simulink model "test_attcontrol"  (R2020b)
settings: Solver=FixedStepAuto  StartTime=0.0  StopTime=N-1  FixedStep=time_step  RelTol=1e-3
values from neighbouring files (symbols this model uses):
  dw_rdt = ones(N,1)    [AttitudeControlTesting.m]
  m_mag = ones(N,1)*[1 1 1]/sqrt(3)    [AttitudeControlTesting.m]
  q_sc = [ones(N/2,1)*[0 0 0 1] ; ones(N/2,1)*[0 sin(pi/4) 0 cos(pi/4)] ]    [AttitudeControlTesting.m]
  time_step = 1    [AttitudeControlTesting.m]    (also in StateTesting.m)
  w_sc = ones(N,1)*deg2rad([0 0 1])    [AttitudeControlTesting.m]
  wr0 = 0    [AttitudeControlTesting.m]
undefined symbols (not defined in the file or in its folder): sim_constants
libraries: vrlib x3
settings Model: Creator=newpo  LastModifiedBy=newpo
settings DataIOCC: ReturnWorkspaceOutputs=off

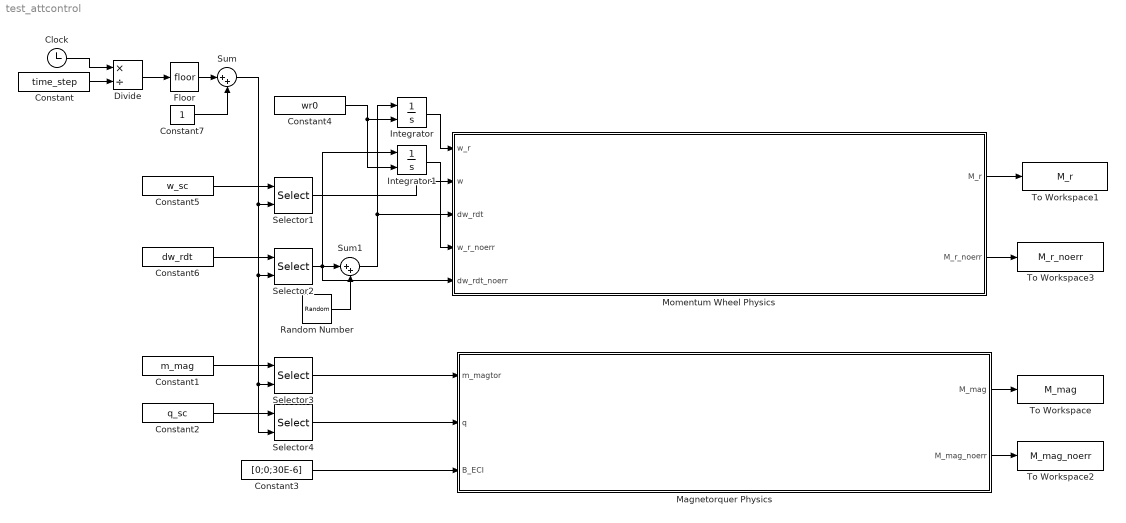
== system test_attcontrol ==
  Clock : Clock
  Constant : Constant  Value=time_step
  Constant1 : Constant  Value=m_mag
  Constant2 : Constant  Value=q_sc
  Constant3 : Constant  Value=[0;0;30E-6]
  Constant4 : Constant  Value=wr0
  Constant5 : Constant  Value=w_sc
  Constant6 : Constant  Value=dw_rdt
  Constant7 : Constant
  Divide : Product  Inputs=*/
  Floor : Rounding
  Integrator : Integrator  InitialConditionSource=external
  Integrator1 : Integrator  InitialConditionSource=external
  Magnetorquer Physics : Subsystem
  Momentum Wheel Physics : Subsystem
  Random Number : RandomNumber  Mean=sim_constants.dw_rdt_bias  Variance=sim_constants.dw_rdt_err  Seed=1  SampleTime=time_step  VectorParams1D=off
  Selector1 : Selector  NumberOfDimensions=2  InputPortWidth=3  IndexOptions=Index vector (port),Index vector (dialog)  Indices=[1 3],[1 2 3]  OutputSizes=1,1
  Selector2 : Selector  InputPortWidth=N  IndexOptions=Index vector (port)  Indices=[1 3]  OutputSizes=1
  Selector3 : Selector  NumberOfDimensions=2  InputPortWidth=3  IndexOptions=Index vector (port),Index vector (dialog)  Indices=[1 3],[1 2 3]  OutputSizes=1,1
  Selector4 : Selector  NumberOfDimensions=2  InputPortWidth=3  IndexOptions=Index vector (port),Index vector (dialog)  Indices=[1 3],[1 2 3 4]  OutputSizes=1,1
  Sum : Sum  Inputs=|++
  Sum1 : Sum  Inputs=|++
  To Workspace : ToWorkspace  VariableName=M_mag  SaveFormat=Timeseries  SampleTime=-1
  To Workspace1 : ToWorkspace  VariableName=M_r  SaveFormat=Timeseries  SampleTime=-1
  To Workspace2 : ToWorkspace  VariableName=M_mag_noerr  SaveFormat=Timeseries  SampleTime=-1
  To Workspace3 : ToWorkspace  VariableName=M_r_noerr  SaveFormat=Timeseries  SampleTime=-1
  wires:
  Selector1/1 -> Momentum Wheel Physics/2(w)
  Constant5/1 -> Selector1/1
  Sum1/1 -> Integrator/1, Momentum Wheel Physics/3(dw_rdt)
  Floor/1 -> Sum/1
  Sum/1 -> Selector4/2, Selector3/2, Selector2/2, Selector1/2
  Constant/1 -> Divide/2
  Clock/1 -> Divide/1
  Divide/1 -> Floor/1
  Constant7/1 -> Sum/2
  Constant6/1 -> Selector2/1
  Integrator/1 -> Momentum Wheel Physics/1(w_r)
  Constant4/1 -> Integrator1/2, Integrator/2
  Selector3/1 -> Magnetorquer Physics/1(m_magtor)
  Constant1/1 -> Selector3/1
  Selector4/1 -> Magnetorquer Physics/2(q)
  Constant2/1 -> Selector4/1
  Constant3/1 -> Magnetorquer Physics/3(B_ECI)
  Magnetorquer Physics/1(M_mag) -> To Workspace/1
  Momentum Wheel Physics/1(M_r) -> To Workspace1/1
  Magnetorquer Physics/2(M_mag_noerr) -> To Workspace2/1
  Momentum Wheel Physics/2(M_r_noerr) -> To Workspace3/1
  Selector2/1 -> Momentum Wheel Physics/5(dw_rdt_noerr), Integrator1/1, Sum1/1
  Random Number/1 -> Sum1/2
  Integrator1/1 -> Momentum Wheel Physics/4(w_r_noerr)

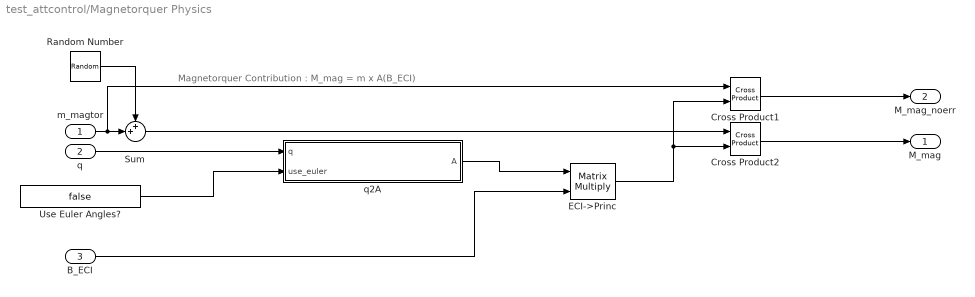
== system test_attcontrol/Magnetorquer Physics ==
  note: Magnetorquer Contribution : M_mag = m x A(B_ECI)
  m_magtor : Inport
  q : Inport  Port=2
  B_ECI : Inport  Port=3
  Cross Product1 : vrlib/Utilities/Cross Product
  Cross Product2 : vrlib/Utilities/Cross Product
  ECI->Princ : Product  Multiplication=Matrix(*)
  Random Number : RandomNumber  Mean=sim_constants.m_magtor_bias  Variance=sim_constants.m_magtor_err  Seed=1  SampleTime=time_step
  Sum : Sum  Inputs=++|
  Use Euler Angles? : Constant  Value=false
  q2A : MATLAB Function  TreatAsAtomicUnit=on
  M_mag : Outport
  M_mag_noerr : Outport  Port=2
  wires:
  ECI->Princ/1 -> Cross Product1/2, Cross Product2/2
  Cross Product2/1 -> M_mag/1
  q2A/1(A) -> ECI->Princ/1
  B_ECI/1 -> ECI->Princ/2
  Use Euler Angles?/1 -> q2A/2(use_euler)
  Sum/1 -> Cross Product2/1
  q/1 -> q2A/1(q)
  m_magtor/1 -> Cross Product1/1, Sum/2
  Random Number/1 -> Sum/1
  Cross Product1/1 -> M_mag_noerr/1

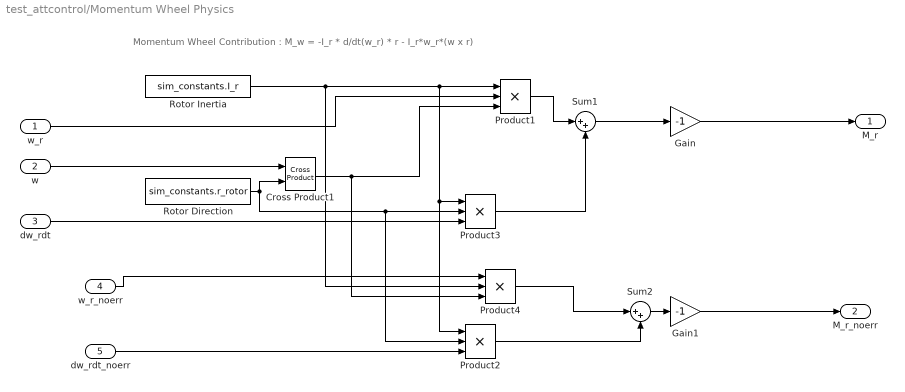
== system test_attcontrol/Momentum Wheel Physics ==
  note: Momentum Wheel Contribution : M_w = -I_r * d/dt(w_r) * r - I_r*w_r*(w x r)
  w_r : Inport
  w : Inport  Port=2
  dw_rdt : Inport  Port=3
  w_r_noerr : Inport  Port=4
  dw_rdt_noerr : Inport  Port=5
  Cross Product1 : vrlib/Utilities/Cross Product
  Gain : Gain  Gain=-1
  Gain1 : Gain  Gain=-1
  Product{1..4} (4 alike) : Product  Inputs=3
  Rotor Direction : Constant  Value=sim_constants.r_rotor
  Rotor Inertia : Constant  Value=sim_constants.I_r
  Sum1 : Sum  Inputs=|++
  Sum2 : Sum  Inputs=|++
  M_r : Outport
  M_r_noerr : Outport  Port=2
  wires:
  Rotor Inertia/1 -> Product4/2, Product2/1, Product3/1, Product1/1
  Product3/1 -> Sum1/2
  Cross Product1/1 -> Product4/3, Product1/3
  Rotor Direction/1 -> Product2/2, Product3/2, Cross Product1/2
  w_r/1 -> Product1/2
  Sum1/1 -> Gain/1
  Product1/1 -> Sum1/1
  dw_rdt/1 -> Product3/3
  Gain/1 -> M_r/1
  w/1 -> Cross Product1/1
  Sum2/1 -> Gain1/1
  Gain1/1 -> M_r_noerr/1
  Product2/1 -> Sum2/2
  w_r_noerr/1 -> Product4/1
  Product4/1 -> Sum2/1
  dw_rdt_noerr/1 -> Product2/3

== matlab function test_attcontrol/Magnetorquer Physics/q2A ==
  data: q input; A output; use_euler input
%% q2A - Calculate cosine matrix from q (or euler angles)
function A = toCosineMatrix(q, use_euler)
    if ~use_euler
        qvec = reshape(q(1:3),3,1);
        skewq = [0 -qvec(3) qvec(2); qvec(3) 0 -qvec(1) ; -qvec(2) qvec(1) 0];
        A = (q(4)^2 - sum(qvec.^2))*eye(3) + 2*qvec*(qvec') - 2*q(4)*skewq ;
    else
        A = [cos(q(1))*cos(q(3))+prod(sin(q(1:3))) sin(q(1))*cos(q(2)) -cos(q(1))*sin(q(3))+sin(q(1))*sin(q(2))*cos(q(3)); 
             (-sin(q(1))*cos(q(3))+cos(q(1))*sin(q(2))*sin(q(3))) (cos(q(1))*cos(q(2))) sin(q(1))*sin(q(3))+cos(q(1))*sin(q(2))*cos(q(3));
             cos(q(2))*sin(q(3)) -sin(q(2)) cos(q(2))*cos(q(3)) ];
        A = A';
    end
end
